simulink model "b_fallschirmTransferBlock"  (R2019b)
settings: Solver=ode45  StartTime=0.0  StopTime=inf  MaxStep=0.1  RelTol=1e-3  EnableMultiTasking=on
model workspace (MAT data in the model file):
  AFS = 30
  AS = 0.5
  cw = 1.3
  g = 9.81
  h0 = 500
  h1 = 47.5029296875
  m = 85
  rho = 1.2
  v0 = 0
settings Model: Creator=Reichl  LastModifiedBy=jakob
settings DataIOCC: SaveFormat=Array  ReturnWorkspaceOutputs=off  OutputSaveName=h
settings OptimizationCC: LifeSpan=inf
settings DebuggingCC: SolverPrmCheckMsg=warning  AllowSymbolicDim=off  SFUnexpectedBacktrackingDiag=warning  SFNoUnconditionalDefaultTransitionDiag=warning  SFExecutionAtInitializationDiag=none  ArithmeticOperatorsInVariantConditions=warning
settings HardwareCC: ProdBitPerPointer=32  ProdBitPerSizeT=32  ProdBitPerPtrDiffT=32  ProdLargestAtomicFloat=None  ProdIntDivRoundTo=Undefined  ProdEndianess=Unspecified  ProdWordSize=32  ProdHWDeviceType=32-bit Generic
settings ModelReferenceCC: PropagateSignalLabelsOutOfModel=off
settings SFSimCC: SimUseLocalCustomCode=off  CustomCodeUndefinedFunction=UseInterfaceOnly
settings RTWCC: RTWUseLocalCustomCode=off
settings CodeAppCC: StateflowObjectComments=on
settings GRTTargetCC: TargetLangStandard=C89/C90 (ANSI)  GeneratePreprocessorConditionals=Disable all
settings ConfigComp: CovMetricSettings=dw  CovHtmlReporting=on  CovSaveCumulativeToWorkspaceVar=on  CovSaveSingleToWorkspaceVar=on  CovExternalEMLEnable=off  CovSFcnEnable=off

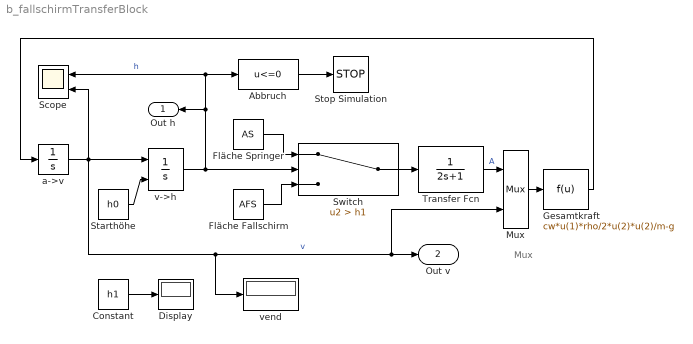
== system b_fallschirmTransferBlock ==
  note: Mux
  Abbruch : Fcn  Expr=u<=0
  Constant : Constant  Value=h1
  Display : Display
  Fläche Fallschirm : Constant  Value=AFS
  Fläche Springer : Constant  Value=AS
  Gesamtkraft : Fcn  Expr=cw*u(1)*rho/2*u(2)*u(2)/m-g
  Mux : Mux  Inputs=2
      settings: DisplayOption=signals
  Scope : Scope  NumInputPorts=2
  Starthöhe : Constant  Value=h0
  Stop Simulation : Stop
  Switch : Switch  Criteria=u2 > Threshold  Threshold=h1  ZeroCross=off
  Transfer Fcn : TransferFcn  Denominator=[2 1]
  a->v : Integrator  InitialCondition=v0
  v->h : Integrator  InitialConditionSource=external
  vend : Display
  Out h : Outport  VectorParamsAs1DForOutWhenUnconnected=off
  Out v : Outport  Port=2  VectorParamsAs1DForOutWhenUnconnected=off
  wires:
  a->v/1 -> vend/1, Mux/2, Out v/1, Scope/2, v->h/1  "v"
  v->h/1 -> Switch/2, Abbruch/1, Scope/1, Out h/1  "h"
  Fläche Springer/1 -> Switch/1
  Fläche Fallschirm/1 -> Switch/3
  Abbruch/1 -> Stop Simulation/1
  Starthöhe/1 -> v->h/2
  Mux/1 -> Gesamtkraft/1
  Gesamtkraft/1 -> a->v/1
  Constant/1 -> Display/1
  Transfer Fcn/1 -> Mux/1  "A"
  Switch/1 -> Transfer Fcn/1
